simulink model "enabledIC"  (R2015a)
settings: Solver=FixedStepDiscrete  StartTime=0.0  StopTime=19.8  FixedStep=0.2  RelTol=1e-3
model workspace (MAT data in the model file):
  already_pp = 1
  input_struct.time = [0; 0.2; 0.4; 0.6; 0.8; 1; 1.2; 1.4; 1.6; 1.8; 2; 2.2; 2.4; 2.6; 2.8; 3; 3.2; 3.4; 3.6; 3.8; 4; 4.2; 4.4; 4.6; 4.8; 5; 5.2; 5.4; 5.6; 5.8; 6; 6.2; 6.4; 6.6; 6.8; 7; 7.2; 7.4; 7.6; 7.8; 8; 8.2; 8.4; 8.6; 8.8; 9; 9.2; 9.4; 9.6; 9.8; 10; 10.2; 10.4; 10.6; 10.8; 11; 11.2; 11.4; 11.6; 11.8; 12; 12.2; 12.4; 12.6; 12.8; 13; 13.2; 13.4; 13.6; 13.8; 14; 14.2; 14.4; 14.6; 14.8; 15; 15.2; 15.4; 15.6; 15.8; 16; 16.2; 16.4; 16.6; 16.8; 17; 17.2; 17.4; 17.6; 17.8; 18; 18.2; 18.4; 18.6; 18.8; 19; 19.2; 19.4; 19.6; 19.8]
  input_struct.signals.name = 'Enable'
  input_struct.signals.values = [0; 1; 0; 0; 0; 1; 0; 0; 0; 0; 0; 0; 1; 1; 1; 1; 1; 0; 1; 0; 0; 1; 0; 0; 0; 0; 0; 0; 1; 1; 0; 1; 1; 0; 0; 1; 1; 0; 1; 0; 0; 1; 1; 1; 1; 1; 1; 0; 0; 1; 0; 1; 0; 0; 0; 1; 0; 0; 1; 0; 1; 1; 1; 0; 1; 1; 1; 0; 1; 0; 0; 1; 1; 1; 1; 0; 1; 0; 0; 0; 0; 0; 0; 1; 0; 1; 0; 1; 1; 1; 1; 0; 1; 0; 0; 0; 0; 1; 0; 1]
  input_struct.signals.dimensions = 1
settings Model: CovMetricSettings=dwe  CovHtmlReporting=off  covSaveCumulativeToWorkspaceVar=off  CovSaveSingleToWorkspaceVar=off  CovExternalEMLEnable=on  Creator=hbourbou  LastModifiedBy=hbourbou
settings DataIOCC: ExternalInput=input_struct  LimitDataPoints=off  LoadExternalInput=on  SaveFormat=Structure  SaveState=on
settings DebuggingCC: SFUnexpectedBacktrackingDiag=error  SFNoUnconditionalDefaultTransitionDiag=error
settings HardwareCC: ProdBitPerPointer=64  ProdLargestAtomicFloat=Float  ProdIntDivRoundTo=Zero  ProdEndianess=LittleEndian  ProdHWDeviceType=Specified
settings ModelReferenceCC: PropagateSignalLabelsOutOfModel=on
settings GRTTargetCC: TargetLangStandard=C99 (ISO)  GeneratePreprocessorConditionals=Use local settings  ExtMode=on

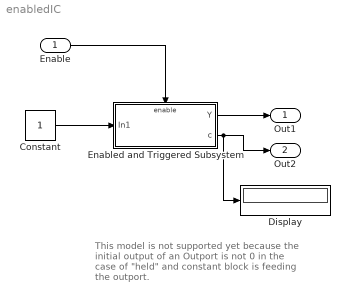
== system enabledIC ==
  note: This model is not supported yet
      |  because the initial output of an Outport
      | is not 0 in the case of "held" and constant
      | block is feeding the outport.
  Enable : Inport  OutDataTypeStr=boolean  PortDimensions=1
  Constant : Constant
  Display : Display
  Enabled and Triggered Subsystem : Subsystem  TreatAsAtomicUnit=on
      settings: MinAlgLoopOccurrences=on
  Out1 : Outport
  Out2 : Outport  Port=2
  wires:
  Constant/1 -> Enabled and Triggered Subsystem/1(In1)
  Enabled and Triggered Subsystem/1(Y) -> Out1/1
  Enable/1 -> Enabled and Triggered Subsystem/Enable
  Enabled and Triggered Subsystem/2(c) -> Display/1, Out2/1

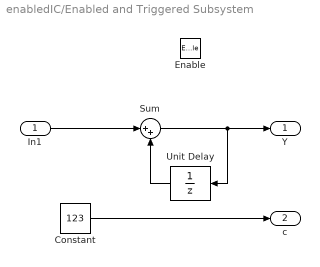
== system enabledIC/Enabled and Triggered Subsystem ==
  In1 : Inport  OutDataTypeStr=double  PortDimensions=1
  Enable : EnablePort  StatesWhenEnabling=reset
  Constant : Constant  Value=123
  Sum : Sum  Inputs=|++
  Unit Delay : UnitDelay  SampleTime=-1
  Y : Outport  InitialOutput=10
  c : Outport  Port=2
  wires:
  In1/1 -> Sum/1
  Sum/1 -> Unit Delay/1, Y/1
  Unit Delay/1 -> Sum/2
  Constant/1 -> c/1
